simulink model "LaserRangeFinderAgent"  (Simulink 6.2)
settings: Solver=ode45  StartTime=0.0  StopTime=10.0  RelTol=1e-3
settings Model: LastModifiedBy=halljf
settings DebuggingCC: SolverPrmCheckMsg=warning

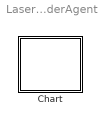
== system LaserRangeFinderAgent ==
  Chart : Stateflow chart

== stateflow chart Chart ==
  state Operation
    \\Sally\PanTilt\PanTiltUnit.Scan()
    \\Sally\PanTilt\PanTiltUnit.HomeLaser()
  state Initial
    \\Sally\PanTilt\PanTiltUnit.InitLaser()
  (default) -> Initial : Start
  Initial -> Operation : Always
